simulink model "subsystem_validation_comp"  (R2020a)
settings: Solver=VariableStepAuto  StartTime=0.0  StopTime=10.0  RelTol=1e-3
values from neighbouring files (symbols this model uses):
  cp_air = gamma_air*cv_air    [Init_Project1.m]    (also in Project2A.m = 980)
  eta_c_max = k(1)    [Project2A.m]
  etaCmin = min(etaC/2)    [Project2A.m]
  gamma_air = EngineMap.airfuel.gamma_air    [Init_Project1.m]    (also in Project2A.m = 1.4)
  m_dot_c_Corr_at = k(2)    [Project2A.m]
  m_dot_cCorr_max = k(2)    [Project2A.m]
  Nc = NcCorr*sqrt(T01/TCref)    [Project2A.m]
  p01 = comp.p01    [Project2A.m]
  p_amb = max(EngineMap.p_af)    [Init_Project1.m]
  pCref = comp.pCref    [Project2A.m]
  PiC = comp.PiC    [Project2A.m]
  PiC_at = k(3)    [Project2A.m]
  Psi_max = k(1)    [Project2A.m]
  Q11 = k(4)    [Project2A.m]
  Q12 = k(5)    [Project2A.m]
  Q22 = k(6)    [Project2A.m]
  rComp = dComp/2    (= 0.028)    [Project2A.m]
  T01 = comp.T01    [Project2A.m]
  TCref = comp.TCref    [Project2A.m]
settings Model: Creator=David Wiman  LastModifiedBy=David Wiman

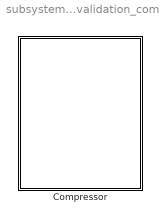
== system subsystem_validation_comp ==
  Compressor : Subsystem

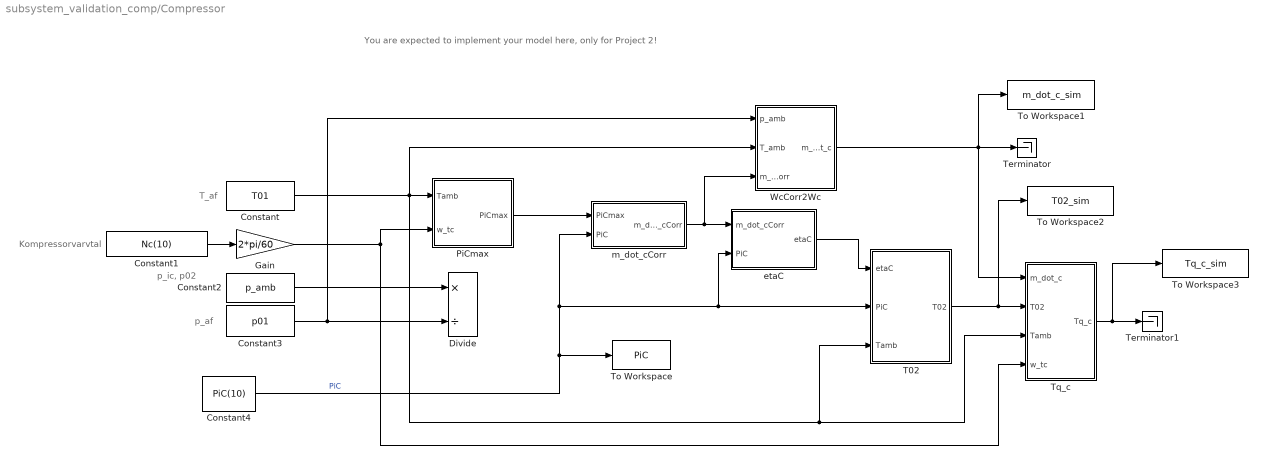
== system subsystem_validation_comp/Compressor ==
  note: T_af
  note: p_af
  note: p_ic, p02
  note: Kompressorvarvtal
  note: You are expected to implement your model here, only for Project 2!
  Constant : Constant  Value=T01
  Constant1 : Constant  Value=Nc(10)
  Constant2 : Constant  Value=p_amb
  Constant3 : Constant  Value=p01
  Constant4 : Constant  Value=PiC(10)
  Divide : Product  Inputs=*/
  Gain : Gain  Gain=2*pi/60
  PiCmax : Subsystem
  T02 : Subsystem
  Terminator : Terminator
  Terminator1 : Terminator
  To Workspace : ToWorkspace  VariableName=PiC  SampleTime=-1
  To Workspace1 : ToWorkspace  VariableName=m_dot_c_sim  SampleTime=-1
  To Workspace2 : ToWorkspace  VariableName=T02_sim  SampleTime=-1
  To Workspace3 : ToWorkspace  VariableName=Tq_c_sim  SampleTime=-1
  Tq_c : Subsystem
  WcCorr2Wc : Subsystem
  etaC : Subsystem
  m_dot_cCorr : Subsystem
  wires:
  Constant1/1 -> Gain/1
  Constant2/1 -> Divide/1
  Constant3/1 -> Divide/2, WcCorr2Wc/1(p_amb)
  Constant/1 -> PiCmax/1(Tamb), WcCorr2Wc/2(T_amb), T02/3(Tamb), Tq_c/3(Tamb)
  WcCorr2Wc/1(m_dot_c) -> Tq_c/1(m_dot_c), To Workspace1/1, Terminator/1
  Constant4/1 -> etaC/2(PiC), T02/2(PiC), m_dot_cCorr/2(PiC), To Workspace/1  "PiC"
  T02/1(T02) -> To Workspace2/1, Tq_c/2(T02)
  Tq_c/1(Tq_c) -> To Workspace3/1, Terminator1/1
  PiCmax/1(PiCmax) -> m_dot_cCorr/1(PiCmax)
  etaC/1(etaC) -> T02/1(etaC)
  Gain/1 -> PiCmax/2(w_tc), Tq_c/4(w_tc)
  m_dot_cCorr/1(m_dot_cCorr) -> WcCorr2Wc/3(m_dot_cCorr), etaC/1(m_dot_cCorr)

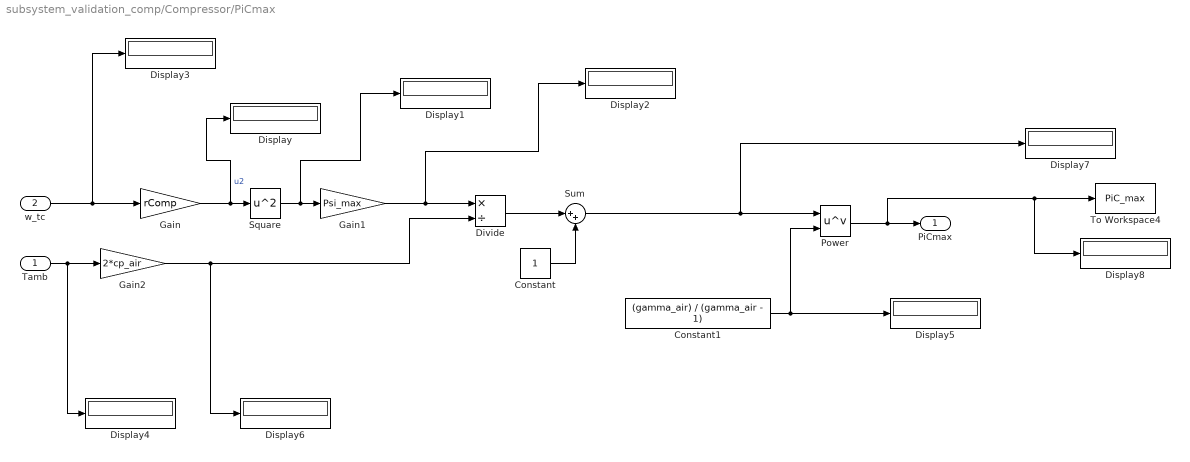
== system subsystem_validation_comp/Compressor/PiCmax ==
  Tamb : Inport
  w_tc : Inport  Port=2
  Constant : Constant
  Constant1 : Constant  Value=(gamma_air) / (gamma_air - 1)
  Display{,1..8} (9 alike) : Display
  Divide : Product  Inputs=*/
  Gain : Gain  Gain=rComp
  Gain1 : Gain  Gain=Psi_max
  Gain2 : Gain  Gain=2*cp_air
  Power : Math  Operator=pow  SaturateOnIntegerOverflow=on
  Square : Math  Operator=square  SaturateOnIntegerOverflow=on
  Sum : Sum  Inputs=|++
  To Workspace4 : ToWorkspace  VariableName=PiC_max  SampleTime=-1
  PiCmax : Outport
  wires:
  w_tc/1 -> Display3/1, Gain/1
  Gain/1 -> Display/1, Square/1  "u2"
  Square/1 -> Display1/1, Gain1/1
  Tamb/1 -> Gain2/1, Display4/1
  Gain1/1 -> Display2/1, Divide/1
  Gain2/1 -> Divide/2, Display6/1
  Constant1/1 -> Power/2, Display5/1
  Power/1 -> Display8/1, To Workspace4/1, PiCmax/1
  Constant/1 -> Sum/2
  Divide/1 -> Sum/1
  Sum/1 -> Display7/1, Power/1

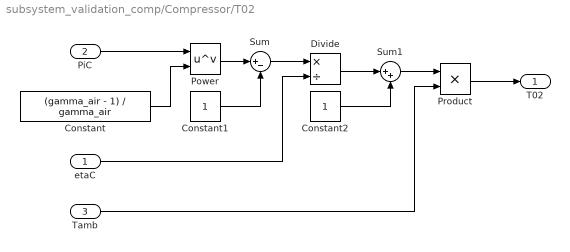
== system subsystem_validation_comp/Compressor/T02 ==
  etaC : Inport
  PiC : Inport  Port=2
  Tamb : Inport  Port=3
  Constant : Constant  Value=(gamma_air - 1) / gamma_air
  Constant1 : Constant
  Constant2 : Constant
  Divide : Product  Inputs=*/
  Power : Math  Operator=pow  SaturateOnIntegerOverflow=on
  Product : Product
  Sum : Sum  Inputs=|+-
  Sum1 : Sum  Inputs=|++
  T02 : Outport
  wires:
  Tamb/1 -> Product/2
  etaC/1 -> Divide/2
  PiC/1 -> Power/1
  Product/1 -> T02/1
  Constant/1 -> Power/2
  Power/1 -> Sum/1
  Constant1/1 -> Sum/2
  Sum/1 -> Divide/1
  Divide/1 -> Sum1/1
  Constant2/1 -> Sum1/2
  Sum1/1 -> Product/1

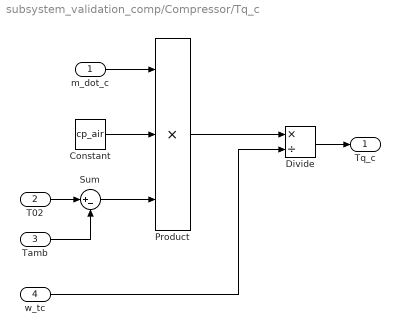
== system subsystem_validation_comp/Compressor/Tq_c ==
  m_dot_c : Inport
  T02 : Inport  Port=2
  Tamb : Inport  Port=3
  w_tc : Inport  Port=4
  Constant : Constant  Value=cp_air
  Divide : Product  Inputs=*/
  Product : Product  Inputs=3
  Sum : Sum  Inputs=|+-
  Tq_c : Outport
  wires:
  Tamb/1 -> Sum/2
  T02/1 -> Sum/1
  m_dot_c/1 -> Product/1
  w_tc/1 -> Divide/2
  Constant/1 -> Product/2
  Sum/1 -> Product/3
  Product/1 -> Divide/1
  Divide/1 -> Tq_c/1

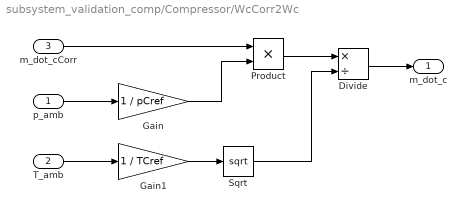
== system subsystem_validation_comp/Compressor/WcCorr2Wc ==
  p_amb : Inport
  T_amb : Inport  Port=2
  m_dot_cCorr : Inport  Port=3
  Divide : Product  Inputs=*/
  Gain : Gain  Gain=1 / pCref
  Gain1 : Gain  Gain=1 / TCref
  Product : Product
  Sqrt : Sqrt  SaturateOnIntegerOverflow=on
  m_dot_c : Outport
  wires:
  Divide/1 -> m_dot_c/1
  T_amb/1 -> Gain1/1
  p_amb/1 -> Gain/1
  m_dot_cCorr/1 -> Product/1
  Gain1/1 -> Sqrt/1
  Gain/1 -> Product/2
  Product/1 -> Divide/1
  Sqrt/1 -> Divide/2

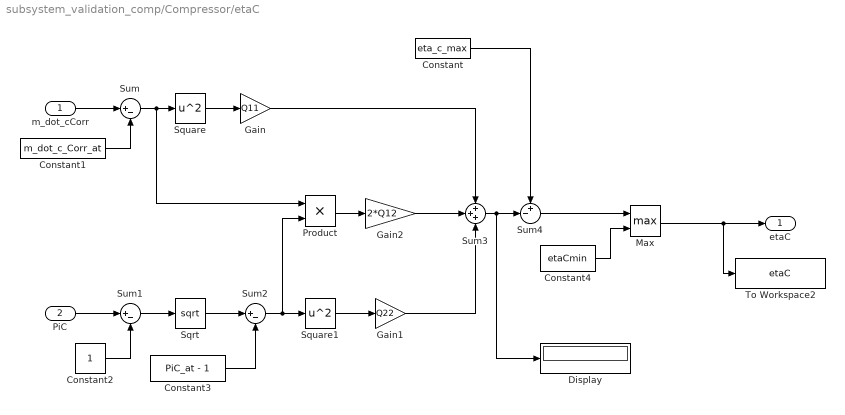
== system subsystem_validation_comp/Compressor/etaC ==
  m_dot_cCorr : Inport
  PiC : Inport  Port=2
  Constant : Constant  Value=eta_c_max
  Constant1 : Constant  Value=m_dot_c_Corr_at
  Constant2 : Constant
  Constant3 : Constant  Value=PiC_at - 1
  Constant4 : Constant  Value=etaCmin
  Display : Display
  Gain : Gain  Gain=Q11
  Gain1 : Gain  Gain=Q22
  Gain2 : Gain  Gain=2*Q12
  Max : MinMax  Function=max  Inputs=2
  Product : Product
  Sqrt : Sqrt  SaturateOnIntegerOverflow=on
  Square : Math  Operator=square  SaturateOnIntegerOverflow=on
  Square1 : Math  Operator=square  SaturateOnIntegerOverflow=on
  Sum : Sum  Inputs=|+-
  Sum1 : Sum  Inputs=|+-
  Sum2 : Sum  Inputs=|+-
  Sum3 : Sum  Inputs=+++
  Sum4 : Sum  Inputs=+-|
  To Workspace2 : ToWorkspace  VariableName=etaC  SampleTime=-1
  etaC : Outport
  wires:
  Sum4/1 -> Max/1
  Constant4/1 -> Max/2
  Max/1 -> To Workspace2/1, etaC/1
  m_dot_cCorr/1 -> Sum/1
  PiC/1 -> Sum1/1
  Constant1/1 -> Sum/2
  Sum/1 -> Product/1, Square/1
  Square/1 -> Gain/1
  Constant2/1 -> Sum1/2
  Sum1/1 -> Sqrt/1
  Sqrt/1 -> Sum2/1
  Sum2/1 -> Product/2, Square1/1
  Square1/1 -> Gain1/1
  Product/1 -> Gain2/1
  Gain2/1 -> Sum3/2
  Gain/1 -> Sum3/1
  Gain1/1 -> Sum3/3
  Sum3/1 -> Display/1, Sum4/2
  Constant/1 -> Sum4/1
  Constant3/1 -> Sum2/2

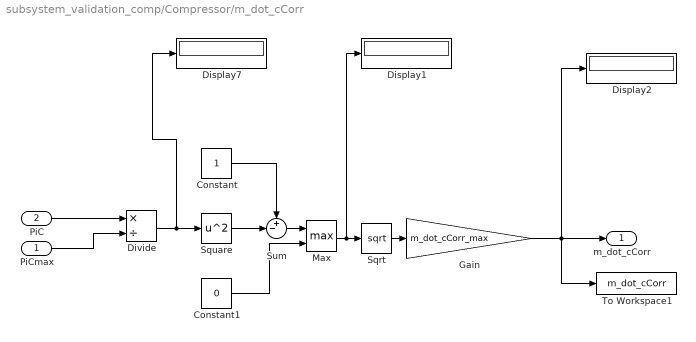
== system subsystem_validation_comp/Compressor/m_dot_cCorr ==
  PiCmax : Inport
  PiC : Inport  Port=2
  Constant : Constant
  Constant1 : Constant  Value=0
  Display1 : Display
  Display2 : Display
  Display7 : Display
  Divide : Product  Inputs=*/
  Gain : Gain  Gain=m_dot_cCorr_max
  Max : MinMax  Function=max  Inputs=2
  Sqrt : Sqrt  SaturateOnIntegerOverflow=on
  Square : Math  Operator=square  SaturateOnIntegerOverflow=on
  Sum : Sum  Inputs=+-|
  To Workspace1 : ToWorkspace  VariableName=m_dot_cCorr  SampleTime=-1
  m_dot_cCorr : Outport
  wires:
  Gain/1 -> Display2/1, To Workspace1/1, m_dot_cCorr/1
  PiCmax/1 -> Divide/2
  PiC/1 -> Divide/1
  Divide/1 -> Display7/1, Square/1
  Square/1 -> Sum/2
  Constant/1 -> Sum/1
  Sqrt/1 -> Gain/1
  Sum/1 -> Max/1
  Max/1 -> Display1/1, Sqrt/1
  Constant1/1 -> Max/2
